simulink model "walkingRobot"  (R2020a)
settings: Solver=ode15s  StartTime=0.0  StopTime=10  EnableMultiTasking=on
PreLoadFcn:
  | robotParameters
  | load('defaultsimulationinputs.mat')
undefined symbols (not defined in the file or in its folder): init_angs_L, init_angs_R, motion_time_constant
libraries: simulink_extras x12, walkingRobotUtils x3, simulink x1
settings Model: SimulationMode=accelerator  Creator=bkim  LastModifiedBy=nikhil
settings DataIOCC: ReturnWorkspaceOutputs=off  OutputSaveName=simout  OutputTimes=0:0.01:10
settings OptimizationCC: LifeSpan=inf
settings DebuggingCC: AllowSymbolicDim=off  PregeneratedLibrarySubsystemCodeDiagnostic=none  SFUnexpectedBacktrackingDiag=warning  SFNoUnconditionalDefaultTransitionDiag=warning  SFExecutionAtInitializationDiag=none  UnitsInconsistencyMsg=none  ArithmeticOperatorsInVariantConditions=warning
settings SFSimCC: SimUseLocalCustomCode=off  CustomCodeUndefinedFunction=UseInterfaceOnly
settings RTWCC: RTWUseLocalCustomCode=off
settings CodeAppCC: StateflowObjectComments=on
settings GRTTargetCC: TargetLangStandard=C89/C90 (ANSI)
settings ConfigComp: CovMetricSettings=dw  CovHtmlReporting=on  CovSaveCumulativeToWorkspaceVar=on  CovSaveSingleToWorkspaceVar=on  CovExternalEMLEnable=off  CovSFcnEnable=off
settings SimscapeCC: SimscapeNormalizeSystem=off  SimscapeLogOpenViewer=on  SimscapeLogLimitData=off  SimscapeLogDataHistory=10000
settings ConfigurationSet: Description=SimMechanics 2G
settings DiagnosticsConfigSet: SimMechanicsRigidlyBoundBlock=none
settings ExplorerConfigSet: InternalSimMechanicsExplorerSettings="<ExplorerConfiguration><canonicalview>default</canonicalview><AnimationSetting><BasePlaybackSpeed>1.0</BasePlaybackSpeed><PlaybackSpeedFactor>1.0</PlaybackSpeedFactor></AnimationSetting><TilePanel><TileInfo><Tiles Columns=\"1\" Count=\"1\" Rows=\"1\"><Column Weight=\"1\"/><Row Weight=\"1\"/><Tile Height=\"1\" Width=\"1\" X=\"0\" Y=\"0\"/></Tiles></TileInfo><SceneInfo><SceneViewer><BGColor><R>0.60000002384185791</R><G>0.60000002384185791</G><B>0.60000002384185791</B></BGColor><Camera><DoPerspective>off</DoPerspective><Position><X>-7.90762128242833562</X><Y>23.8081096481694914</Y><Z>5.91146841204722939</Z></Position><Center><X>-0.406277996262525587</X><Y>0.615564294304502546</Y><Z>-0.277309600720595628</Z></Center><Up><X>0.182671955115720652</X><Y>-0.197900690545468771</Y><Z>0.963050504125213092</Z></Up><ViewLimDist>1</ViewLimDist><YLim>2.56954837368236522</YLim><XLim>3.29520786810192234</XLim></Camera></SceneViewer></SceneInfo></TilePanel><MechEditorPanel><Cameras/><GfxPanelCameraMap/><VideoCreator><PlaybackSpeedRatio>1.0</PlaybackSpeedRatio><FrameRate>30</FrameRate><VideoFormat>Motion JPEG AVI</VideoFormat><FrameSize>auto</FrameSize></VideoCreator></MechEditorPanel></ExplorerConfiguration>"

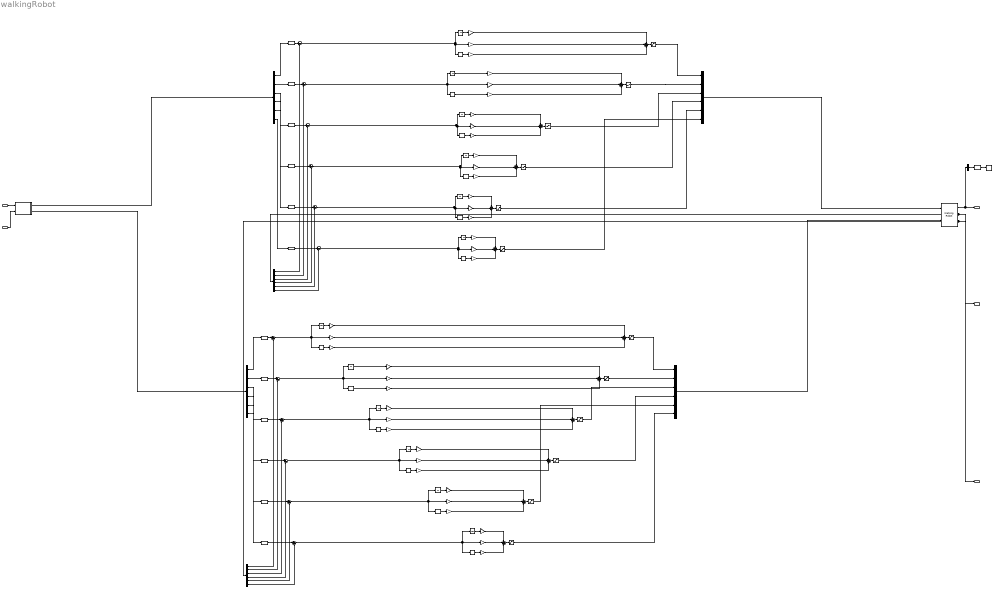
== system walkingRobot ==
  note: Controller6
  note: Controller11
  note: Controller10
  note: Controller9
  note: Controller8
  note: Controller7
  note: Controller5
  note: Controller4
  note: Controller3
  note: Controller2
  note: Controller1
  note: Controller
  note: PID Controllers L
  note: PID Controllers R
  note: Walking Robot Model
      |
      | Copyright 2017-2019 The MathWorks, Inc.
  footR : Inport
  footL : Inport  Port=2
  Bus Creator : BusCreator  Inputs=6
  Bus Creator1 : BusCreator  Inputs=6
  Bus Selector : BusSelector  OutputSignals=Z
  Bus Selector1 : BusSelector  OutputSignals=ankleroll_angle,anklepitch_angle,knee_angle,hippitch_angle,hiproll_angle,hipyaw_angle
  Bus Selector2 : BusSelector  OutputSignals=ankleroll_angle,anklepitch_angle,knee_angle,hippitch_angle,hiproll_angle,hipyaw_angle
  Bus Selector3 : BusSelector  OutputSignals=ankle roll,ankle pitch,knee,hip pitch,hip roll,hip yaw
  Bus Selector4 : BusSelector  OutputSignals=ankle roll,ankle pitch,knee,hip pitch,hip roll,hip yaw
  Derivative{,1..11} (12 alike) : Derivative
  Detect Fallen Robot : simulink/Logic and Bit Operations/Compare To Constant  relop=<=  const=0.3  OutDataTypeStr=boolean
  Gain{1,4,7,10,13,16,19,22,25,28,31,34} (12 alike) : Gain  Gain=0.02175
  Gain{2,5,8,11,14,17,20,23,26,29,32,35} (12 alike) : Gain  Gain=0.495
  Gain{3,6,9,12,15,18,21,24,27,30,33,36} (12 alike) : Gain  Gain=0.115
  Integrator{,1..11} (12 alike) : Integrator
  Inverse Kinematics : Subsystem
  Low-Pass Filter : simulink_extras/Additional Linear/Transfer Fcn (with initial outputs)  N=[(1/motion_time_constant)^2]  D=[1 2/motion_time_constant (1/motion_time_constant)^2]  Y0=init_angs_R(6)  U0=init_angs_R(6)
  Low-Pass Filter1 : simulink_extras/Additional Linear/Transfer Fcn (with initial outputs)  N=[(1/motion_time_constant)^2]  D=[1 2/motion_time_constant (1/motion_time_constant)^2]  Y0=init_angs_R(5)  U0=init_angs_R(5)
  Low-Pass Filter10 : simulink_extras/Additional Linear/Transfer Fcn (with initial outputs)  N=[(1/motion_time_constant)^2]  D=[1 2/motion_time_constant (1/motion_time_constant)^2]  Y0=init_angs_L(2)  U0=init_angs_L(2)
  Low-Pass Filter11 : simulink_extras/Additional Linear/Transfer Fcn (with initial outputs)  N=[(1/motion_time_constant)^2]  D=[1 2/motion_time_constant (1/motion_time_constant)^2]  Y0=init_angs_L(1)  U0=init_angs_L(1)
  Low-Pass Filter2 : simulink_extras/Additional Linear/Transfer Fcn (with initial outputs)  N=[(1/motion_time_constant)^2]  D=[1 2/motion_time_constant (1/motion_time_constant)^2]  Y0=init_angs_R(4)  U0=init_angs_R(4)
  Low-Pass Filter3 : simulink_extras/Additional Linear/Transfer Fcn (with initial outputs)  N=[(1/motion_time_constant)^2]  D=[1 2/motion_time_constant (1/motion_time_constant)^2]  Y0=init_angs_R(3)  U0=init_angs_R(3)
  Low-Pass Filter4 : simulink_extras/Additional Linear/Transfer Fcn (with initial outputs)  N=[(1/motion_time_constant)^2]  D=[1 2/motion_time_constant (1/motion_time_constant)^2]  Y0=init_angs_R(2)  U0=init_angs_R(2)
  Low-Pass Filter5 : simulink_extras/Additional Linear/Transfer Fcn (with initial outputs)  N=[(1/motion_time_constant)^2]  D=[1 2/motion_time_constant (1/motion_time_constant)^2]  Y0=init_angs_R(1)  U0=init_angs_R(1)
  Low-Pass Filter6 : simulink_extras/Additional Linear/Transfer Fcn (with initial outputs)  N=[(1/motion_time_constant)^2]  D=[1 2/motion_time_constant (1/motion_time_constant)^2]  Y0=init_angs_L(6)  U0=init_angs_L(6)
  Low-Pass Filter7 : simulink_extras/Additional Linear/Transfer Fcn (with initial outputs)  N=[(1/motion_time_constant)^2]  D=[1 2/motion_time_constant (1/motion_time_constant)^2]  Y0=init_angs_L(5)  U0=init_angs_L(5)
  Low-Pass Filter8 : simulink_extras/Additional Linear/Transfer Fcn (with initial outputs)  N=[(1/motion_time_constant)^2]  D=[1 2/motion_time_constant (1/motion_time_constant)^2]  Y0=init_angs_L(4)  U0=init_angs_L(4)
  Low-Pass Filter9 : simulink_extras/Additional Linear/Transfer Fcn (with initial outputs)  N=[(1/motion_time_constant)^2]  D=[1 2/motion_time_constant (1/motion_time_constant)^2]  Y0=init_angs_L(3)  U0=init_angs_L(3)
  Saturation{,1..11} (12 alike) : Saturate  UpperLimit=15  LowerLimit=-15
  Stop Simulation : Stop
  Sum{1..12} (12 alike) : Sum  Inputs=|+-
  Sum{13..24} (12 alike) : Sum  Inputs=+++
  Walking Robot : walkingRobotUtils/Walking Robot  SystemSampleTime=-1  Latency=0  AutoFrameSizeCalculation=off
  measBody : Outport  VectorParamsAs1DForOutWhenUnconnected=off
  measR : Outport  Port=2  VectorParamsAs1DForOutWhenUnconnected=off
  measL : Outport  Port=3  VectorParamsAs1DForOutWhenUnconnected=off
  wires:
  Walking Robot/3 -> measL/1, Bus Selector2/1  "measL"
  Walking Robot/2 -> measR/1, Bus Selector1/1  "measR"
  Bus Creator/1 -> Walking Robot/1
  Bus Creator1/1 -> Walking Robot/2
  footR/1 -> Inverse Kinematics/1(footR)  "footR"
  footL/1 -> Inverse Kinematics/2(footL)  "footL"
  Walking Robot/1 -> Bus Selector/1, measBody/1  "measBody"
  Bus Selector/1 -> Detect Fallen Robot/1  "<Z>"
  Detect Fallen Robot/1 -> Stop Simulation/1
  Inverse Kinematics/1(refR) -> Bus Selector4/1  "refR"
  Inverse Kinematics/2(refL) -> Bus Selector3/1  "refL"
  Low-Pass Filter5/1 -> Sum8/1
  Low-Pass Filter/1 -> Sum6/1
  Bus Selector4/6 -> Low-Pass Filter5/1  "<hip yaw>"
  Saturation4/1 -> Bus Creator/5  "hip roll"
  Bus Selector4/2 -> Low-Pass Filter1/1  "<ankle pitch>"
  Bus Selector4/4 -> Low-Pass Filter3/1  "<hip pitch>"
  Saturation1/1 -> Bus Creator/2  "ankle pitch"
  Saturation5/1 -> Bus Creator/6  "hip yaw"
  Saturation2/1 -> Bus Creator/3  "knee"
  Bus Selector4/3 -> Low-Pass Filter2/1  "<knee>"
  Bus Selector4/1 -> Low-Pass Filter/1  "<ankle roll>"
  Bus Selector1/3 -> Sum2/2  "<knee_angle>"
  Bus Selector4/5 -> Low-Pass Filter4/1  "<hip roll>"
  Saturation/1 -> Bus Creator/1  "ankle roll"
  Low-Pass Filter3/1 -> Sum3/1
  Bus Selector1/6 -> Sum8/2  "<hipyaw_angle>"
  Saturation3/1 -> Bus Creator/4  "hip pitch"
  Bus Selector1/5 -> Sum7/2  "<hiproll_angle>"
  Low-Pass Filter1/1 -> Sum1/1
  Bus Selector1/1 -> Sum6/2  "<ankleroll_angle>"
  Low-Pass Filter2/1 -> Sum2/1
  Low-Pass Filter4/1 -> Sum7/1
  Bus Selector1/4 -> Sum3/2  "<hippitch_angle>"
  Bus Selector1/2 -> Sum1/2  "<anklepitch_angle>"
  Saturation7/1 -> Bus Creator1/2  "ankle pitch"
  Saturation10/1 -> Bus Creator1/5  "hip roll"
  Saturation9/1 -> Bus Creator1/4  "hip pitch"
  Saturation8/1 -> Bus Creator1/3  "knee"
  Saturation6/1 -> Bus Creator1/1  "ankle roll"
  Bus Selector2/2 -> Sum4/2  "<anklepitch_angle>"
  Bus Selector2/4 -> Sum9/2  "<hippitch_angle>"
  Low-Pass Filter10/1 -> Sum11/1
  Low-Pass Filter8/1 -> Sum5/1
  Bus Selector2/1 -> Sum10/2  "<ankleroll_angle>"
  Low-Pass Filter7/1 -> Sum4/1
  Bus Selector2/5 -> Sum11/2  "<hiproll_angle>"
  Bus Selector2/6 -> Sum12/2  "<hipyaw_angle>"
  Low-Pass Filter9/1 -> Sum9/1
  Bus Selector3/5 -> Low-Pass Filter10/1  "<hip roll>"
  Bus Selector2/3 -> Sum5/2  "<knee_angle>"
  Bus Selector3/1 -> Low-Pass Filter6/1  "<ankle roll>"
  Bus Selector3/3 -> Low-Pass Filter8/1  "<knee>"
  Saturation11/1 -> Bus Creator1/6  "hip yaw"
  Bus Selector3/4 -> Low-Pass Filter9/1  "<hip pitch>"
  Bus Selector3/2 -> Low-Pass Filter7/1  "<ankle pitch>"
  Bus Selector3/6 -> Low-Pass Filter11/1  "<hip yaw>"
  Low-Pass Filter6/1 -> Sum10/1
  Low-Pass Filter11/1 -> Sum12/1
  Integrator/1 -> Gain1/1
  Sum13/1 -> Saturation/1
  Derivative/1 -> Gain3/1
  Sum6/1 -> Derivative/1, Gain2/1, Integrator/1  "err"
  Gain3/1 -> Sum13/3  "gain3"
  Gain2/1 -> Sum13/2  "gain2"
  Gain1/1 -> Sum13/1  "gain1"
  Integrator1/1 -> Gain4/1
  Sum14/1 -> Saturation1/1
  Derivative1/1 -> Gain6/1
  Sum1/1 -> Derivative1/1, Gain5/1, Integrator1/1  "err"
  Gain6/1 -> Sum14/3  "gain6"
  Gain5/1 -> Sum14/2  "gain5"
  Gain4/1 -> Sum14/1  "gain4"
  Integrator2/1 -> Gain7/1
  Sum15/1 -> Saturation2/1
  Derivative2/1 -> Gain9/1
  Sum2/1 -> Derivative2/1, Gain8/1, Integrator2/1  "err"
  Gain9/1 -> Sum15/3  "gain9"
  Gain8/1 -> Sum15/2  "gain8"
  Gain7/1 -> Sum15/1  "gain7"
  Integrator3/1 -> Gain10/1
  Sum16/1 -> Saturation3/1
  Derivative3/1 -> Gain12/1
  Sum3/1 -> Derivative3/1, Gain11/1, Integrator3/1  "err"
  Gain12/1 -> Sum16/3  "gain12"
  Gain11/1 -> Sum16/2  "gain11"
  Gain10/1 -> Sum16/1  "gain10"
  Integrator4/1 -> Gain13/1
  Sum17/1 -> Saturation4/1
  Derivative4/1 -> Gain15/1
  Sum7/1 -> Derivative4/1, Gain14/1, Integrator4/1  "err"
  Gain15/1 -> Sum17/3  "gain15"
  Gain14/1 -> Sum17/2  "gain14"
  Gain13/1 -> Sum17/1  "gain13"
  Integrator5/1 -> Gain16/1
  Sum18/1 -> Saturation5/1
  Derivative5/1 -> Gain18/1
  Sum8/1 -> Derivative5/1, Gain17/1, Integrator5/1  "err"
  Gain18/1 -> Sum18/3  "gain18"
  Gain17/1 -> Sum18/2  "gain17"
  Gain16/1 -> Sum18/1  "gain16"
  Integrator6/1 -> Gain19/1
  Sum19/1 -> Saturation6/1
  Derivative6/1 -> Gain21/1
  Sum10/1 -> Derivative6/1, Gain20/1, Integrator6/1  "err"
  Gain21/1 -> Sum19/3  "gain21"
  Gain20/1 -> Sum19/2  "gain20"
  Gain19/1 -> Sum19/1  "gain19"
  Integrator7/1 -> Gain22/1
  Sum20/1 -> Saturation7/1
  Derivative7/1 -> Gain24/1
  Sum4/1 -> Derivative7/1, Gain23/1, Integrator7/1  "err"
  Gain24/1 -> Sum20/3  "gain24"
  Gain23/1 -> Sum20/2  "gain23"
  Gain22/1 -> Sum20/1  "gain22"
  Integrator8/1 -> Gain25/1
  Sum21/1 -> Saturation8/1
  Derivative8/1 -> Gain27/1
  Sum5/1 -> Derivative8/1, Gain26/1, Integrator8/1  "err"
  Gain27/1 -> Sum21/3  "gain27"
  Gain26/1 -> Sum21/2  "gain26"
  Gain25/1 -> Sum21/1  "gain25"
  Integrator9/1 -> Gain28/1
  Sum22/1 -> Saturation9/1
  Derivative9/1 -> Gain30/1
  Sum9/1 -> Derivative9/1, Gain29/1, Integrator9/1  "err"
  Gain30/1 -> Sum22/3  "gain30"
  Gain29/1 -> Sum22/2  "gain29"
  Gain28/1 -> Sum22/1  "gain28"
  Integrator10/1 -> Gain31/1
  Sum23/1 -> Saturation10/1
  Derivative10/1 -> Gain33/1
  Sum11/1 -> Derivative10/1, Gain32/1, Integrator10/1  "err"
  Gain33/1 -> Sum23/3  "gain33"
  Gain32/1 -> Sum23/2  "gain32"
  Gain31/1 -> Sum23/1  "gain31"
  Integrator11/1 -> Gain34/1
  Sum24/1 -> Saturation11/1
  Derivative11/1 -> Gain36/1
  Sum12/1 -> Derivative11/1, Gain35/1, Integrator11/1  "err"
  Gain36/1 -> Sum24/3  "gain36"
  Gain35/1 -> Sum24/2  "gain35"
  Gain34/1 -> Sum24/1  "gain34"

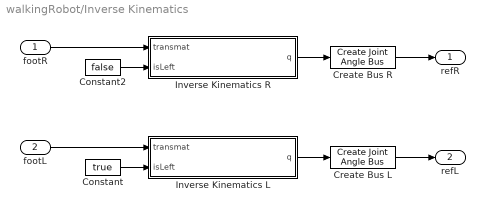
== system walkingRobot/Inverse Kinematics ==
  footR : Inport
  footL : Inport  Port=2
  Constant : Constant  Value=true
  Constant2 : Constant  Value=false
  Create Bus L : walkingRobotUtils/Create Joint Angle Bus  SystemSampleTime=-1  Latency=0  AutoFrameSizeCalculation=off
  Create Bus R : walkingRobotUtils/Create Joint Angle Bus  SystemSampleTime=-1  Latency=0  AutoFrameSizeCalculation=off
  Inverse Kinematics L : MATLAB Function  TreatAsAtomicUnit=on
  Inverse Kinematics R : MATLAB Function  TreatAsAtomicUnit=on
  refR : Outport
  refL : Outport  Port=2
  wires:
  footR/1 -> Inverse Kinematics R/1(transmat)
  Inverse Kinematics L/1(q) -> Create Bus L/1
  Constant2/1 -> Inverse Kinematics R/2(isLeft)
  Create Bus R/1 -> refR/1
  Create Bus L/1 -> refL/1
  Constant/1 -> Inverse Kinematics L/2(isLeft)
  Inverse Kinematics R/1(q) -> Create Bus R/1
  footL/1 -> Inverse Kinematics L/1(transmat)

== matlab function walkingRobot/Inverse Kinematics/Inverse Kinematics R ==
  data: transmat input; q output; isLeft input
function q = inverseKinematics(transmat, isLeft)
q = invKinBody2Foot(transmat, isLeft);

== matlab function walkingRobot/Inverse Kinematics/Inverse Kinematics L ==
  data: transmat input; q output; isLeft input
function q = inverseKinematics(transmat, isLeft)
q = invKinBody2Foot(transmat, isLeft);
